simulink model "c00009M_harness"  (R2018a)
settings: Solver=FixedStepAuto  StartTime=0.0  StopTime=300  FixedStep=0.1  RelTol=1e-3
undefined symbols (not defined in the file): A1, hmax, PriorityTank, R1, R2, sigbuilder_block
(part 1 of 29)
settings Model: Creator=aarrieta  LastModifiedBy=umarkiegi

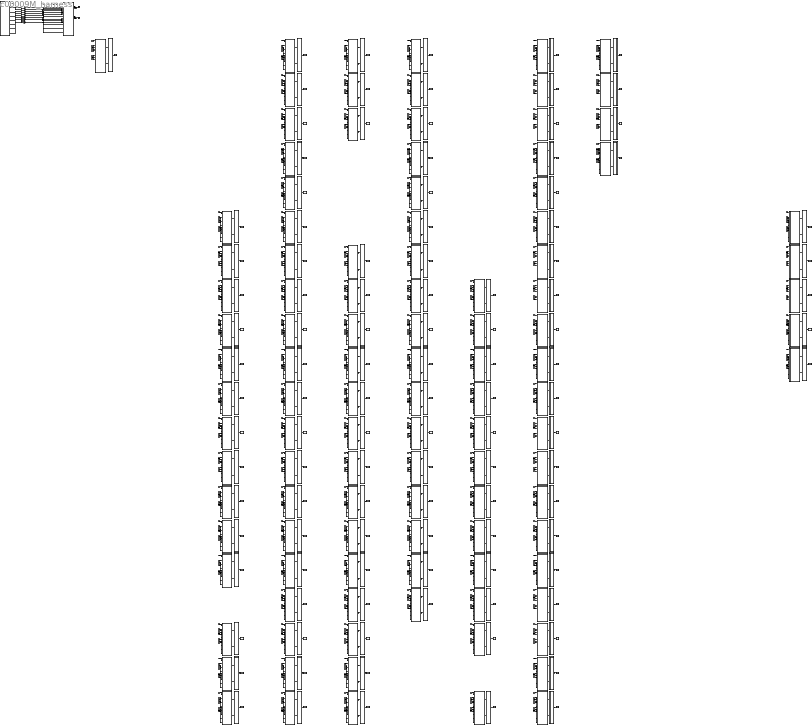
== system c00009M_harness ==
  CPSUT : Subsystem
  Eval : Subsystem
  Eval100 : Subsystem
  Eval101 : Subsystem
  Eval102 : Subsystem
  Eval103 : Subsystem
  Eval104 : Subsystem
  Eval105 : Subsystem
  Eval106 : Subsystem
  Eval107 : Subsystem
  Eval108 : Subsystem
  Eval109 : Subsystem
  Eval110 : Subsystem
  Eval111 : Subsystem
  Eval112 : Subsystem
  Eval113 : Subsystem
  Eval114 : Subsystem
  Eval115 : Subsystem
  Eval116 : Subsystem
  Eval127 : Subsystem
  Eval128 : Subsystem
  Eval129 : Subsystem
  Eval130 : Subsystem
  Eval131 : Subsystem
  Eval132 : Subsystem
  Eval133 : Subsystem
  Eval134 : Subsystem
  Eval135 : Subsystem
  Eval136 : Subsystem
  Eval137 : Subsystem
  Eval139 : Subsystem
  Eval140 : Subsystem
  Eval141 : Subsystem
  Eval142 : Subsystem
  Eval143 : Subsystem
  Eval144 : Subsystem
  Eval145 : Subsystem
  Eval146 : Subsystem
  Eval147 : Subsystem
  Eval148 : Subsystem
  Eval149 : Subsystem
  Eval150 : Subsystem
  Eval151 : Subsystem
  Eval152 : Subsystem
  Eval153 : Subsystem
  Eval154 : Subsystem
  Eval155 : Subsystem
  Eval156 : Subsystem
  Eval157 : Subsystem
  Eval158 : Subsystem
  Eval159 : Subsystem
  Eval160 : Subsystem
  Eval161 : Subsystem
  Eval162 : Subsystem
  Eval163 : Subsystem
  Eval225 : Subsystem
  Eval226 : Subsystem
  Eval227 : Subsystem
  Eval228 : Subsystem
  Eval229 : Subsystem
  Eval45 : Subsystem
  Eval46 : Subsystem
  Eval47 : Subsystem
  Eval48 : Subsystem
  Eval49 : Subsystem
  Eval50 : Subsystem
  Eval51 : Subsystem
  Eval52 : Subsystem
  Eval53 : Subsystem
  Eval54 : Subsystem
  Eval55 : Subsystem
  Eval57 : Subsystem
  Eval58 : Subsystem
  Eval59 : Subsystem
  Eval60 : Subsystem
  Eval61 : Subsystem
  Eval62 : Subsystem
  Eval63 : Subsystem
  Eval64 : Subsystem
  Eval65 : Subsystem
  Eval66 : Subsystem
  Eval67 : Subsystem
  Eval68 : Subsystem
  Eval69 : Subsystem
  Eval70 : Subsystem
  Eval71 : Subsystem
  Eval72 : Subsystem
  Eval73 : Subsystem
  Eval74 : Subsystem
  Eval75 : Subsystem
  Eval76 : Subsystem
  Eval77 : Subsystem
  Eval78 : Subsystem
  Eval79 : Subsystem
  Eval80 : Subsystem
  Eval81 : Subsystem
  Eval82 : Subsystem
  Eval86 : Subsystem
  Eval87 : Subsystem
  Eval88 : Subsystem
  Eval89 : Subsystem
  Eval90 : Subsystem
  Eval91 : Subsystem
  Eval92 : Subsystem
  Eval93 : Subsystem
  Eval94 : Subsystem
  Eval95 : Subsystem
  Eval96 : Subsystem
  Eval97 : Subsystem
  Eval98 : Subsystem
  Eval99 : Subsystem
  Inputs : Subsystem  Tag=STV Subsys  LoadFcn=sigbuilder_block('load');  StartFcn=sigbuilder_block('start');  StopFcn=sigbuilder_block('stop');  ClipboardFcn=sigbuilder_block('clipboard');  mask(Sigbuilder block){tuvar=[0:10]}
      mask init:
      | if ~strcmp(get_param(bdroot(gcb),'SimulationStatus'),'stopped'),tuvar = sigbuilder_block('maskInit'); end
      settings: CopyFcn=sigbuilder_block('copy');  DeleteFcn=sigbuilder_block('delete');  ModelCloseFcn=sigbuilder_block('modelClose');  PreSaveFcn=sigbuilder_block('preSave');  PauseFcn=sigbuilder_block('pause');  ContinueFcn=sigbuilder_block('continue');  NameChangeFcn=sigbuilder_block('namechange');  OpenFcn=sigbuilder_block('open',[276.75 163.5 675.75 486.75 ]);  CloseFcn=sigbuilder_block('close');
      mask Display: plot(0, 0, 100, 100,[2, 2, 32, 32, 2], [68, 8, 8, 68, 68],[32, 2], [38, 38], [32, 19, 2],[53, 60, 44], [32, 17, 17, 2],[16, 16, 31, 31]);txt = getActiveGroup(gcbh);text(2, 100, txt,'verticalAlignment', 'top');
  M001 : Subsystem
  M046 : Subsystem
  M047 : Subsystem
  M048 : Subsystem
  M049 : Subsystem
  M050 : Subsystem
  M051 : Subsystem
  M052 : Subsystem
  M053 : Subsystem
  M054 : Subsystem
  M055 : Subsystem
  M056 : Subsystem
  M058 : Subsystem
  M059 : Subsystem
  M060 : Subsystem
  M061 : Subsystem
  M062 : Subsystem
  M063 : Subsystem
  M064 : Subsystem
  M065 : Subsystem
  M066 : Subsystem
  M067 : Subsystem
  M068 : Subsystem
  M069 : Subsystem
  M070 : Subsystem
  M071 : Subsystem
  M072 : Subsystem
  M073 : Subsystem
  M074 : Subsystem
  M075 : Subsystem
  M076 : Subsystem
  M077 : Subsystem
  M078 : Subsystem
  M079 : Subsystem
  M080 : Subsystem
  M081 : Subsystem
  M082 : Subsystem
  M083 : Subsystem
  M087 : Subsystem
  M088 : Subsystem
  M089 : Subsystem
  M090 : Subsystem
  M091 : Subsystem
  M092 : Subsystem
  M093 : Subsystem
  M094 : Subsystem
  M095 : Subsystem
  M096 : Subsystem
  M097 : Subsystem
  M098 : Subsystem
  M099 : Subsystem
  M100 : Subsystem
  M101 : Subsystem
  M102 : Subsystem
  M103 : Subsystem
  M104 : Subsystem
  M105 : Subsystem
  M106 : Subsystem
  M107 : Subsystem
  M108 : Subsystem
  M109 : Subsystem
  M110 : Subsystem
  M111 : Subsystem
  M112 : Subsystem
  M113 : Subsystem
  M114 : Subsystem
  M115 : Subsystem
  M116 : Subsystem
  M117 : Subsystem
  M128 : Subsystem
  M129 : Subsystem
  M130 : Subsystem
  M131 : Subsystem
  M132 : Subsystem
  M133 : Subsystem
  M134 : Subsystem
  M135 : Subsystem
  M136 : Subsystem
  M137 : Subsystem
  M138 : Subsystem
  M140 : Subsystem
  M141 : Subsystem
  M142 : Subsystem
  M143 : Subsystem
  M144 : Subsystem
  M145 : Subsystem
  M146 : Subsystem
  M147 : Subsystem
  M148 : Subsystem
  M149 : Subsystem
  M150 : Subsystem
  M151 : Subsystem
  M152 : Subsystem
  M153 : Subsystem
  M154 : Subsystem
  M155 : Subsystem
  M156 : Subsystem
  M157 : Subsystem
  M158 : Subsystem
  M159 : Subsystem
  M160 : Subsystem
  M161 : Subsystem
  M162 : Subsystem
  M163 : Subsystem
  M164 : Subsystem
  M226 : Subsystem
  M227 : Subsystem
  M228 : Subsystem
  M229 : Subsystem
  M230 : Subsystem
  To Workspace : ToWorkspace  VariableName=mutant001  SampleTime=-1
  To Workspace100 : ToWorkspace  VariableName=mutant101  SampleTime=-1
  To Workspace101 : ToWorkspace  VariableName=mutant102  SampleTime=-1
  To Workspace102 : ToWorkspace  VariableName=mutant103  SampleTime=-1
  To Workspace103 : ToWorkspace  VariableName=mutant104  SampleTime=-1
  To Workspace104 : ToWorkspace  VariableName=mutant105  SampleTime=-1
  To Workspace105 : ToWorkspace  VariableName=mutant106  SampleTime=-1
  To Workspace106 : ToWorkspace  VariableName=mutant107  SampleTime=-1
  To Workspace107 : ToWorkspace  VariableName=mutant108  SampleTime=-1
  To Workspace108 : ToWorkspace  VariableName=mutant109  SampleTime=-1
  To Workspace109 : ToWorkspace  VariableName=mutant110  SampleTime=-1
  To Workspace110 : ToWorkspace  VariableName=mutant111  SampleTime=-1
  To Workspace111 : ToWorkspace  VariableName=mutant112  SampleTime=-1
  To Workspace112 : ToWorkspace  VariableName=mutant113  SampleTime=-1
  To Workspace113 : ToWorkspace  VariableName=mutant114  SampleTime=-1
  To Workspace114 : ToWorkspace  VariableName=mutant115  SampleTime=-1
  To Workspace115 : ToWorkspace  VariableName=mutant116  SampleTime=-1
  To Workspace116 : ToWorkspace  VariableName=mutant117  SampleTime=-1
  To Workspace127 : ToWorkspace  VariableName=mutant128  SampleTime=-1
  To Workspace128 : ToWorkspace  VariableName=mutant129  SampleTime=-1
  To Workspace129 : ToWorkspace  VariableName=mutant130  SampleTime=-1
  To Workspace130 : ToWorkspace  VariableName=mutant131  SampleTime=-1
  To Workspace131 : ToWorkspace  VariableName=mutant132  SampleTime=-1
  To Workspace132 : ToWorkspace  VariableName=mutant133  SampleTime=-1
  To Workspace133 : ToWorkspace  VariableName=mutant134  SampleTime=-1
  To Workspace134 : ToWorkspace  VariableName=mutant135  SampleTime=-1
  To Workspace135 : ToWorkspace  VariableName=mutant136  SampleTime=-1
  To Workspace136 : ToWorkspace  VariableName=mutant137  SampleTime=-1
  To Workspace137 : ToWorkspace  VariableName=mutant138  SampleTime=-1
  To Workspace139 : ToWorkspace  VariableName=mutant140  SampleTime=-1
  To Workspace140 : ToWorkspace  VariableName=mutant141  SampleTime=-1
  To Workspace141 : ToWorkspace  VariableName=mutant142  SampleTime=-1
  To Workspace142 : ToWorkspace  VariableName=mutant143  SampleTime=-1
  To Workspace143 : ToWorkspace  VariableName=mutant144  SampleTime=-1
  To Workspace144 : ToWorkspace  VariableName=mutant145  SampleTime=-1
  To Workspace145 : ToWorkspace  VariableName=mutant146  SampleTime=-1
  To Workspace146 : ToWorkspace  VariableName=mutant147  SampleTime=-1
  To Workspace147 : ToWorkspace  VariableName=mutant148  SampleTime=-1
  To Workspace148 : ToWorkspace  VariableName=mutant149  SampleTime=-1
  To Workspace149 : ToWorkspace  VariableName=mutant150  SampleTime=-1
  To Workspace150 : ToWorkspace  VariableName=mutant151  SampleTime=-1
  To Workspace151 : ToWorkspace  VariableName=mutant152  SampleTime=-1
  To Workspace152 : ToWorkspace  VariableName=mutant153  SampleTime=-1
  To Workspace153 : ToWorkspace  VariableName=mutant154  SampleTime=-1
  To Workspace154 : ToWorkspace  VariableName=mutant155  SampleTime=-1
  To Workspace155 : ToWorkspace  VariableName=mutant156  SampleTime=-1
  To Workspace156 : ToWorkspace  VariableName=mutant157  SampleTime=-1
  To Workspace157 : ToWorkspace  VariableName=mutant158  SampleTime=-1
  To Workspace158 : ToWorkspace  VariableName=mutant159  SampleTime=-1
  To Workspace159 : ToWorkspace  VariableName=mutant160  SampleTime=-1
  To Workspace160 : ToWorkspace  VariableName=mutant161  SampleTime=-1
  To Workspace161 : ToWorkspace  VariableName=mutant162  SampleTime=-1
  To Workspace162 : ToWorkspace  VariableName=mutant163  SampleTime=-1
  To Workspace163 : ToWorkspace  VariableName=mutant164  SampleTime=-1
  To Workspace225 : ToWorkspace  VariableName=mutant226  SampleTime=-1
  To Workspace226 : ToWorkspace  VariableName=mutant227  SampleTime=-1
  To Workspace227 : ToWorkspace  VariableName=mutant228  SampleTime=-1
  To Workspace228 : ToWorkspace  VariableName=mutant229  SampleTime=-1
  To Workspace229 : ToWorkspace  VariableName=mutant230  SampleTime=-1
  To Workspace45 : ToWorkspace  VariableName=mutant046  SampleTime=-1
  To Workspace46 : ToWorkspace  VariableName=mutant047  SampleTime=-1
  To Workspace47 : ToWorkspace  VariableName=mutant048  SampleTime=-1
  To Workspace48 : ToWorkspace  VariableName=mutant049  SampleTime=-1
  To Workspace49 : ToWorkspace  VariableName=mutant050  SampleTime=-1
  To Workspace50 : ToWorkspace  VariableName=mutant051  SampleTime=-1
  To Workspace51 : ToWorkspace  VariableName=mutant052  SampleTime=-1
  To Workspace52 : ToWorkspace  VariableName=mutant053  SampleTime=-1
  To Workspace53 : ToWorkspace  VariableName=mutant054  SampleTime=-1
  To Workspace54 : ToWorkspace  VariableName=mutant055  SampleTime=-1
  To Workspace55 : ToWorkspace  VariableName=mutant056  SampleTime=-1
  To Workspace57 : ToWorkspace  VariableName=mutant058  SampleTime=-1
  To Workspace58 : ToWorkspace  VariableName=mutant059  SampleTime=-1
  To Workspace59 : ToWorkspace  VariableName=mutant060  SampleTime=-1
  To Workspace60 : ToWorkspace  VariableName=mutant061  SampleTime=-1
  To Workspace61 : ToWorkspace  VariableName=mutant062  SampleTime=-1
  To Workspace62 : ToWorkspace  VariableName=mutant063  SampleTime=-1
  To Workspace63 : ToWorkspace  VariableName=mutant064  SampleTime=-1
  To Workspace64 : ToWorkspace  VariableName=mutant065  SampleTime=-1
  To Workspace65 : ToWorkspace  VariableName=mutant066  SampleTime=-1
  To Workspace66 : ToWorkspace  VariableName=mutant067  SampleTime=-1
  To Workspace67 : ToWorkspace  VariableName=mutant068  SampleTime=-1
  To Workspace68 : ToWorkspace  VariableName=mutant069  SampleTime=-1
  To Workspace69 : ToWorkspace  VariableName=mutant070  SampleTime=-1
  To Workspace70 : ToWorkspace  VariableName=mutant071  SampleTime=-1
  To Workspace71 : ToWorkspace  VariableName=mutant072  SampleTime=-1
  To Workspace72 : ToWorkspace  VariableName=mutant073  SampleTime=-1
  To Workspace73 : ToWorkspace  VariableName=mutant074  SampleTime=-1
  To Workspace74 : ToWorkspace  VariableName=mutant075  SampleTime=-1
  To Workspace75 : ToWorkspace  VariableName=mutant076  SampleTime=-1
  To Workspace76 : ToWorkspace  VariableName=mutant077  SampleTime=-1
  To Workspace77 : ToWorkspace  VariableName=mutant078  SampleTime=-1
  To Workspace78 : ToWorkspace  VariableName=mutant079  SampleTime=-1
  To Workspace79 : ToWorkspace  VariableName=mutant080  SampleTime=-1
  To Workspace80 : ToWorkspace  VariableName=mutant081  SampleTime=-1
  To Workspace81 : ToWorkspace  VariableName=mutant082  SampleTime=-1
  To Workspace82 : ToWorkspace  VariableName=mutant083  SampleTime=-1
  To Workspace86 : ToWorkspace  VariableName=mutant087  SampleTime=-1
  To Workspace87 : ToWorkspace  VariableName=mutant088  SampleTime=-1
  To Workspace88 : ToWorkspace  VariableName=mutant089  SampleTime=-1
  To Workspace89 : ToWorkspace  VariableName=mutant090  SampleTime=-1
  To Workspace90 : ToWorkspace  VariableName=mutant091  SampleTime=-1
  To Workspace91 : ToWorkspace  VariableName=mutant092  SampleTime=-1
  To Workspace92 : ToWorkspace  VariableName=mutant093  SampleTime=-1
  To Workspace93 : ToWorkspace  VariableName=mutant094  SampleTime=-1
  To Workspace94 : ToWorkspace  VariableName=mutant095  SampleTime=-1
  To Workspace95 : ToWorkspace  VariableName=mutant096  SampleTime=-1
  To Workspace96 : ToWorkspace  VariableName=mutant097  SampleTime=-1
  To Workspace97 : ToWorkspace  VariableName=mutant098  SampleTime=-1
  To Workspace98 : ToWorkspace  VariableName=mutant099  SampleTime=-1
  To Workspace99 : ToWorkspace  VariableName=mutant100  SampleTime=-1
  dtc_CT1 : DataTypeConversion
  dtc_CT2 : DataTypeConversion
  dtc_EB1 : DataTypeConversion
  dtc_EB2 : DataTypeConversion
  dtc_MR1 : DataTypeConversion
  dtc_MR2 : DataTypeConversion
  dtc_T1 : DataTypeConversion
  dtc_T2 : DataTypeConversion
  LL1 : Outport
  LL2 : Outport  Port=2
  tag scope: out1=global, out2=global
  wires:
  CPSUT/1(LL1) -> [out1], LL1/1
  CPSUT/2(LL2) -> [out2], LL2/1
  [in1] -> M001/1(CT1)
  [in4] -> M001/2(MR1)
  [in5] -> M001/3(T1)
  [in6] -> M001/4(EB1)
  [in7] -> M001/5(CT2)
  [in10] -> M001/6(MR2)
  [in11] -> M001/7(T2)
  [in12] -> M001/8(EB2)
  Eval/1(Out1) -> To Workspace/1
  M001/1(LL1) -> Eval/1(In1)
  M001/2(LL2) -> Eval/2(In2)
  [in1] -> M046/1(CT1)
  [in4] -> M046/2(MR1)
  [in5] -> M046/3(T1)
  [in6] -> M046/4(EB1)
  [in7] -> M046/5(CT2)
  [in10] -> M046/6(MR2)
  [in11] -> M046/7(T2)
  [in12] -> M046/8(EB2)
  M046/1(LL1) -> Eval45/1(In1)
  M046/2(LL2) -> Eval45/2(In2)
  Eval45/1(Out1) -> To Workspace45/1
  [in1] -> M047/1(CT1)
  [in4] -> M047/2(MR1)
  [in5] -> M047/3(T1)
  [in6] -> M047/4(EB1)
  [in7] -> M047/5(CT2)
  [in10] -> M047/6(MR2)
  [in11] -> M047/7(T2)
  [in12] -> M047/8(EB2)
  M047/1(LL1) -> Eval46/1(In1)
  M047/2(LL2) -> Eval46/2(In2)
  Eval46/1(Out1) -> To Workspace46/1
  [in1] -> M048/1(CT1)
  [in4] -> M048/2(MR1)
  [in5] -> M048/3(T1)
  [in6] -> M048/4(EB1)
  [in7] -> M048/5(CT2)
  [in10] -> M048/6(MR2)
  [in11] -> M048/7(T2)
  [in12] -> M048/8(EB2)
  M048/1(LL1) -> Eval47/1(In1)
  M048/2(LL2) -> Eval47/2(In2)
  Eval47/1(Out1) -> To Workspace47/1
  [in1] -> M049/1(CT1)
  [in4] -> M049/2(MR1)
  [in5] -> M049/3(T1)
  [in6] -> M049/4(EB1)
  [in7] -> M049/5(CT2)
  [in10] -> M049/6(MR2)
  [in11] -> M049/7(T2)
  [in12] -> M049/8(EB2)
  M049/1(LL1) -> Eval48/1(In1)
  M049/2(LL2) -> Eval48/2(In2)
  Eval48/1(Out1) -> To Workspace48/1
  [in1] -> M050/1(CT1)
  [in4] -> M050/2(MR1)
  [in5] -> M050/3(T1)
  [in6] -> M050/4(EB1)
  [in7] -> M050/5(CT2)
  [in10] -> M050/6(MR2)
  [in11] -> M050/7(T2)
  [in12] -> M050/8(EB2)
  M050/1(LL1) -> Eval49/1(In1)
  M050/2(LL2) -> Eval49/2(In2)
  Eval49/1(Out1) -> To Workspace49/1
  [in1] -> M051/1(CT1)
  [in4] -> M051/2(MR1)
  [in5] -> M051/3(T1)
  [in6] -> M051/4(EB1)
  [in7] -> M051/5(CT2)
  [in10] -> M051/6(MR2)
  [in11] -> M051/7(T2)
  [in12] -> M051/8(EB2)
  M051/1(LL1) -> Eval50/1(In1)
  M051/2(LL2) -> Eval50/2(In2)
  Eval50/1(Out1) -> To Workspace50/1
  [in1] -> M052/1(CT1)
  [in4] -> M052/2(MR1)
  [in5] -> M052/3(T1)
  [in6] -> M052/4(EB1)
  [in7] -> M052/5(CT2)
  [in10] -> M052/6(MR2)
  [in11] -> M052/7(T2)
  [in12] -> M052/8(EB2)
  M052/1(LL1) -> Eval51/1(In1)
  M052/2(LL2) -> Eval51/2(In2)
  Eval51/1(Out1) -> To Workspace51/1
  [in1] -> M053/1(CT1)
  [in4] -> M053/2(MR1)
  [in5] -> M053/3(T1)
  [in6] -> M053/4(EB1)
  [in7] -> M053/5(CT2)
  [in10] -> M053/6(MR2)
  [in11] -> M053/7(T2)
  [in12] -> M053/8(EB2)
  M053/1(LL1) -> Eval52/1(In1)
  M053/2(LL2) -> Eval52/2(In2)
  Eval52/1(Out1) -> To Workspace52/1
  [in1] -> M054/1(CT1)
  [in4] -> M054/2(MR1)
  [in5] -> M054/3(T1)
  [in6] -> M054/4(EB1)
  [in7] -> M054/5(CT2)
  [in10] -> M054/6(MR2)
  [in11] -> M054/7(T2)
  [in12] -> M054/8(EB2)
  M054/1(LL1) -> Eval53/1(In1)
  M054/2(LL2) -> Eval53/2(In2)
  Eval53/1(Out1) -> To Workspace53/1
  [in1] -> M055/1(CT1)
  [in4] -> M055/2(MR1)
  [in5] -> M055/3(T1)
  [in6] -> M055/4(EB1)
  [in7] -> M055/5(CT2)
  [in10] -> M055/6(MR2)
  [in11] -> M055/7(T2)
  [in12] -> M055/8(EB2)
  M055/1(LL1) -> Eval54/1(In1)
  M055/2(LL2) -> Eval54/2(In2)
  Eval54/1(Out1) -> To Workspace54/1
  [in1] -> M056/1(CT1)
  [in4] -> M056/2(MR1)
  [in5] -> M056/3(T1)
  [in6] -> M056/4(EB1)
  [in7] -> M056/5(CT2)
  [in10] -> M056/6(MR2)
  [in11] -> M056/7(T2)
  [in12] -> M056/8(EB2)
  M056/1(LL1) -> Eval55/1(In1)
  M056/2(LL2) -> Eval55/2(In2)
  Eval55/1(Out1) -> To Workspace55/1
  [in1] -> M058/1(CT1)
  [in4] -> M058/2(MR1)
  [in5] -> M058/3(T1)
  [in6] -> M058/4(EB1)
  [in7] -> M058/5(CT2)
  [in10] -> M058/6(MR2)
  [in11] -> M058/7(T2)
  [in12] -> M058/8(EB2)
  M058/1(LL1) -> Eval57/1(In1)
  M058/2(LL2) -> Eval57/2(In2)
  Eval57/1(Out1) -> To Workspace57/1
  [in1] -> M059/1(CT1)
  [in4] -> M059/2(MR1)
  [in5] -> M059/3(T1)
  [in6] -> M059/4(EB1)
  [in7] -> M059/5(CT2)
  [in10] -> M059/6(MR2)
  [in11] -> M059/7(T2)
  [in12] -> M059/8(EB2)
  M059/1(LL1) -> Eval58/1(In1)
  M059/2(LL2) -> Eval58/2(In2)
  Eval58/1(Out1) -> To Workspace58/1
  [in1] -> M060/1(CT1)
  [in4] -> M060/2(MR1)
  [in5] -> M060/3(T1)
  [in6] -> M060/4(EB1)
  [in7] -> M060/5(CT2)
  [in10] -> M060/6(MR2)
  [in11] -> M060/7(T2)
  [in12] -> M060/8(EB2)
  M060/1(LL1) -> Eval59/1(In1)
  M060/2(LL2) -> Eval59/2(In2)
  Eval59/1(Out1) -> To Workspace59/1
  [in1] -> M061/1(CT1)
  [in4] -> M061/2(MR1)
  [in5] -> M061/3(T1)
  [in6] -> M061/4(EB1)
  [in7] -> M061/5(CT2)
  [in10] -> M061/6(MR2)
  [in11] -> M061/7(T2)
  [in12] -> M061/8(EB2)
  M061/1(LL1) -> Eval60/1(In1)
  M061/2(LL2) -> Eval60/2(In2)
  Eval60/1(Out1) -> To Workspace60/1
  [in1] -> M062/1(CT1)
  [in4] -> M062/2(MR1)
  [in5] -> M062/3(T1)
  [in6] -> M062/4(EB1)
  [in7] -> M062/5(CT2)
  [in10] -> M062/6(MR2)
  [in11] -> M062/7(T2)
  [in12] -> M062/8(EB2)
  M062/1(LL1) -> Eval61/1(In1)
  M062/2(LL2) -> Eval61/2(In2)
  Eval61/1(Out1) -> To Workspace61/1
  [in1] -> M063/1(CT1)
  [in4] -> M063/2(MR1)
  [in5] -> M063/3(T1)
  [in6] -> M063/4(EB1)
  [in7] -> M063/5(CT2)
  [in10] -> M063/6(MR2)
  [in11] -> M063/7(T2)
  [in12] -> M063/8(EB2)
  M063/1(LL1) -> Eval62/1(In1)
  M063/2(LL2) -> Eval62/2(In2)
  Eval62/1(Out1) -> To Workspace62/1
  [in1] -> M064/1(CT1)
  [in4] -> M064/2(MR1)
  [in5] -> M064/3(T1)
  [in6] -> M064/4(EB1)
  [in7] -> M064/5(CT2)
  [in10] -> M064/6(MR2)
  [in11] -> M064/7(T2)
  [in12] -> M064/8(EB2)
  M064/1(LL1) -> Eval63/1(In1)
  M064/2(LL2) -> Eval63/2(In2)
  Eval63/1(Out1) -> To Workspace63/1
  [in1] -> M065/1(CT1)
  [in4] -> M065/2(MR1)
  [in5] -> M065/3(T1)
  [in6] -> M065/4(EB1)
  [in7] -> M065/5(CT2)
  [in10] -> M065/6(MR2)
  [in11] -> M065/7(T2)
  [in12] -> M065/8(EB2)
  M065/1(LL1) -> Eval64/1(In1)
  M065/2(LL2) -> Eval64/2(In2)
  Eval64/1(Out1) -> To Workspace64/1
  [in1] -> M066/1(CT1)
  [in4] -> M066/2(MR1)
  [in5] -> M066/3(T1)
  [in6] -> M066/4(EB1)
  [in7] -> M066/5(CT2)
  [in10] -> M066/6(MR2)
  [in11] -> M066/7(T2)
  [in12] -> M066/8(EB2)
  M066/1(LL1) -> Eval65/1(In1)
  M066/2(LL2) -> Eval65/2(In2)
  Eval65/1(Out1) -> To Workspace65/1
  [in1] -> M067/1(CT1)
  [in4] -> M067/2(MR1)
  [in5] -> M067/3(T1)
  [in6] -> M067/4(EB1)
  [in7] -> M067/5(CT2)
  [in10] -> M067/6(MR2)
  [in11] -> M067/7(T2)
  [in12] -> M067/8(EB2)
  M067/1(LL1) -> Eval66/1(In1)
  M067/2(LL2) -> Eval66/2(In2)
  Eval66/1(Out1) -> To Workspace66/1
  [in1] -> M068/1(CT1)
  [in4] -> M068/2(MR1)
  [in5] -> M068/3(T1)
  [in6] -> M068/4(EB1)
  [in7] -> M068/5(CT2)
  [in10] -> M068/6(MR2)
  [in11] -> M068/7(T2)
  [in12] -> M068/8(EB2)
  M068/1(LL1) -> Eval67/1(In1)
  M068/2(LL2) -> Eval67/2(In2)
  Eval67/1(Out1) -> To Workspace67/1
  [in1] -> M069/1(CT1)
  [in4] -> M069/2(MR1)
  [in5] -> M069/3(T1)
  [in6] -> M069/4(EB1)
  [in7] -> M069/5(CT2)
  [in10] -> M069/6(MR2)
  [in11] -> M069/7(T2)
  [in12] -> M069/8(EB2)
  M069/1(LL1) -> Eval68/1(In1)
  M069/2(LL2) -> Eval68/2(In2)
  Eval68/1(Out1) -> To Workspace68/1
  [in1] -> M070/1(CT1)
  [in4] -> M070/2(MR1)
  [in5] -> M070/3(T1)
  [in6] -> M070/4(EB1)
  [in7] -> M070/5(CT2)
  [in10] -> M070/6(MR2)
  [in11] -> M070/7(T2)
  [in12] -> M070/8(EB2)
  M070/1(LL1) -> Eval69/1(In1)
  M070/2(LL2) -> Eval69/2(In2)
  Eval69/1(Out1) -> To Workspace69/1
  [in1] -> M071/1(CT1)
  [in4] -> M071/2(MR1)
  [in5] -> M071/3(T1)
  [in6] -> M071/4(EB1)
  [in7] -> M071/5(CT2)
  [in10] -> M071/6(MR2)
  [in11] -> M071/7(T2)
  [in12] -> M071/8(EB2)
  M071/1(LL1) -> Eval70/1(In1)
  M071/2(LL2) -> Eval70/2(In2)
  Eval70/1(Out1) -> To Workspace70/1
  [in1] -> M072/1(CT1)
  [in4] -> M072/2(MR1)
  [in5] -> M072/3(T1)
  [in6] -> M072/4(EB1)
  [in7] -> M072/5(CT2)
  [in10] -> M072/6(MR2)
  [in11] -> M072/7(T2)
  [in12] -> M072/8(EB2)
  M072/1(LL1) -> Eval71/1(In1)
  M072/2(LL2) -> Eval71/2(In2)
  Eval71/1(Out1) -> To Workspace71/1
  [in1] -> M073/1(CT1)
  [in4] -> M073/2(MR1)
  [in5] -> M073/3(T1)
  [in6] -> M073/4(EB1)
  [in7] -> M073/5(CT2)
  [in10] -> M073/6(MR2)
  [in11] -> M073/7(T2)
  [in12] -> M073/8(EB2)
  M073/1(LL1) -> Eval72/1(In1)
  M073/2(LL2) -> Eval72/2(In2)
  Eval72/1(Out1) -> To Workspace72/1
  [in1] -> M074/1(CT1)
  [in4] -> M074/2(MR1)
  [in5] -> M074/3(T1)
  [in6] -> M074/4(EB1)
  [in7] -> M074/5(CT2)
  [in10] -> M074/6(MR2)
  [in11] -> M074/7(T2)
  [in12] -> M074/8(EB2)
  M074/1(LL1) -> Eval73/1(In1)
  M074/2(LL2) -> Eval73/2(In2)
  Eval73/1(Out1) -> To Workspace73/1
  [in1] -> M075/1(CT1)
  [in4] -> M075/2(MR1)
  [in5] -> M075/3(T1)
  [in6] -> M075/4(EB1)
  [in7] -> M075/5(CT2)
  [in10] -> M075/6(MR2)
  [in11] -> M075/7(T2)
  [in12] -> M075/8(EB2)
  M075/1(LL1) -> Eval74/1(In1)
  M075/2(LL2) -> Eval74/2(In2)
  Eval74/1(Out1) -> To Workspace74/1
  [in1] -> M076/1(CT1)
  [in4] -> M076/2(MR1)
  [in5] -> M076/3(T1)
  [in6] -> M076/4(EB1)
  [in7] -> M076/5(CT2)
  [in10] -> M076/6(MR2)
  [in11] -> M076/7(T2)
  [in12] -> M076/8(EB2)
  M076/1(LL1) -> Eval75/1(In1)
  M076/2(LL2) -> Eval75/2(In2)
  Eval75/1(Out1) -> To Workspace75/1
  [in1] -> M077/1(CT1)
  [in4] -> M077/2(MR1)
  [in5] -> M077/3(T1)
  [in6] -> M077/4(EB1)
  [in7] -> M077/5(CT2)
  [in10] -> M077/6(MR2)
  [in11] -> M077/7(T2)
  [in12] -> M077/8(EB2)
  M077/1(LL1) -> Eval76/1(In1)
  M077/2(LL2) -> Eval76/2(In2)
  Eval76/1(Out1) -> To Workspace76/1
  [in1] -> M078/1(CT1)
  [in4] -> M078/2(MR1)
  [in5] -> M078/3(T1)
  [in6] -> M078/4(EB1)
  [in7] -> M078/5(CT2)
  [in10] -> M078/6(MR2)
  [in11] -> M078/7(T2)
  [in12] -> M078/8(EB2)
  M078/1(LL1) -> Eval77/1(In1)
  M078/2(LL2) -> Eval77/2(In2)
  Eval77/1(Out1) -> To Workspace77/1
  [in1] -> M079/1(CT1)
  [in4] -> M079/2(MR1)
  [in5] -> M079/3(T1)
  [in6] -> M079/4(EB1)
  [in7] -> M079/5(CT2)
  [in10] -> M079/6(MR2)
  [in11] -> M079/7(T2)
  [in12] -> M079/8(EB2)
  M079/1(LL1) -> Eval78/1(In1)
  M079/2(LL2) -> Eval78/2(In2)
  Eval78/1(Out1) -> To Workspace78/1
  [in1] -> M080/1(CT1)
  [in4] -> M080/2(MR1)
  [in5] -> M080/3(T1)
  [in6] -> M080/4(EB1)
  [in7] -> M080/5(CT2)
  [in10] -> M080/6(MR2)
  [in11] -> M080/7(T2)
  [in12] -> M080/8(EB2)
  M080/1(LL1) -> Eval79/1(In1)
  M080/2(LL2) -> Eval79/2(In2)
  Eval79/1(Out1) -> To Workspace79/1
  [in1] -> M081/1(CT1)
  [in4] -> M081/2(MR1)
  [in5] -> M081/3(T1)
  [in6] -> M081/4(EB1)
  [in7] -> M081/5(CT2)
  [in10] -> M081/6(MR2)
  [in11] -> M081/7(T2)
  [in12] -> M081/8(EB2)
  M081/1(LL1) -> Eval80/1(In1)
  M081/2(LL2) -> Eval80/2(In2)
  Eval80/1(Out1) -> To Workspace80/1
  [in1] -> M082/1(CT1)
  [in4] -> M082/2(MR1)
  [in5] -> M082/3(T1)
  [in6] -> M082/4(EB1)
  [in7] -> M082/5(CT2)
  [in10] -> M082/6(MR2)
  [in11] -> M082/7(T2)
  [in12] -> M082/8(EB2)
  M082/1(LL1) -> Eval81/1(In1)
  M082/2(LL2) -> Eval81/2(In2)
  Eval81/1(Out1) -> To Workspace81/1
  [in1] -> M083/1(CT1)
  [in4] -> M083/2(MR1)
  [in5] -> M083/3(T1)
  [in6] -> M083/4(EB1)
  [in7] -> M083/5(CT2)
  [in10] -> M083/6(MR2)
  [in11] -> M083/7(T2)
  [in12] -> M083/8(EB2)
  M083/1(LL1) -> Eval82/1(In1)
  M083/2(LL2) -> Eval82/2(In2)
  Eval82/1(Out1) -> To Workspace82/1
  [in1] -> M087/1(CT1)
  [in4] -> M087/2(MR1)
  [in5] -> M087/3(T1)
  [in6] -> M087/4(EB1)
  [in7] -> M087/5(CT2)
  [in10] -> M087/6(MR2)
  [in11] -> M087/7(T2)
  [in12] -> M087/8(EB2)
  M087/1(LL1) -> Eval86/1(In1)
  M087/2(LL2) -> Eval86/2(In2)
  Eval86/1(Out1) -> To Workspace86/1
  [in1] -> M088/1(CT1)
  [in4] -> M088/2(MR1)
  [in5] -> M088/3(T1)
  [in6] -> M088/4(EB1)
  [in7] -> M088/5(CT2)
  [in10] -> M088/6(MR2)
  [in11] -> M088/7(T2)
  [in12] -> M088/8(EB2)
  M088/1(LL1) -> Eval87/1(In1)
  M088/2(LL2) -> Eval87/2(In2)
  Eval87/1(Out1) -> To Workspace87/1
  [in1] -> M089/1(CT1)
  [in4] -> M089/2(MR1)
  [in5] -> M089/3(T1)
  [in6] -> M089/4(EB1)
  [in7] -> M089/5(CT2)
  [in10] -> M089/6(MR2)
  [in11] -> M089/7(T2)
  [in12] -> M089/8(EB2)
  M089/1(LL1) -> Eval88/1(In1)
  M089/2(LL2) -> Eval88/2(In2)
  Eval88/1(Out1) -> To Workspace88/1
  [in1] -> M090/1(CT1)
  [in4] -> M090/2(MR1)
  [in5] -> M090/3(T1)
  [in6] -> M090/4(EB1)
  [in7] -> M090/5(CT2)
  [in10] -> M090/6(MR2)
  [in11] -> M090/7(T2)
  [in12] -> M090/8(EB2)
  M090/1(LL1) -> Eval89/1(In1)
  M090/2(LL2) -> Eval89/2(In2)
  Eval89/1(Out1) -> To Workspace89/1
  [in1] -> M091/1(CT1)
  [in4] -> M091/2(MR1)
  [in5] -> M091/3(T1)
  [in6] -> M091/4(EB1)
  [in7] -> M091/5(CT2)
  [in10] -> M091/6(MR2)
  [in11] -> M091/7(T2)
  [in12] -> M091/8(EB2)
  M091/1(LL1) -> Eval90/1(In1)
  M091/2(LL2) -> Eval90/2(In2)
  Eval90/1(Out1) -> To Workspace90/1
  [in1] -> M092/1(CT1)
  [in4] -> M092/2(MR1)
  [in5] -> M092/3(T1)
  [in6] -> M092/4(EB1)
  [in7] -> M092/5(CT2)
  [in10] -> M092/6(MR2)
  [in11] -> M092/7(T2)
  [in12] -> M092/8(EB2)
  M092/1(LL1) -> Eval91/1(In1)
  M092/2(LL2) -> Eval91/2(In2)
  Eval91/1(Out1) -> To Workspace91/1
  [in1] -> M093/1(CT1)
  [in4] -> M093/2(MR1)
  [in5] -> M093/3(T1)
  [in6] -> M093/4(EB1)
  [in7] -> M093/5(CT2)
  [in10] -> M093/6(MR2)
  [in11] -> M093/7(T2)
  [in12] -> M093/8(EB2)
  M093/1(LL1) -> Eval92/1(In1)
  M093/2(LL2) -> Eval92/2(In2)
  Eval92/1(Out1) -> To Workspace92/1
  [in1] -> M094/1(CT1)
  [in4] -> M094/2(MR1)
  [in5] -> M094/3(T1)
  [in6] -> M094/4(EB1)
  [in7] -> M094/5(CT2)
  [in10] -> M094/6(MR2)
  [in11] -> M094/7(T2)
  [in12] -> M094/8(EB2)
  M094/1(LL1) -> Eval93/1(In1)
  M094/2(LL2) -> Eval93/2(In2)
  Eval93/1(Out1) -> To Workspace93/1
  [in1] -> M095/1(CT1)
  [in4] -> M095/2(MR1)
  [in5] -> M095/3(T1)
  [in6] -> M095/4(EB1)
  [in7] -> M095/5(CT2)
  [in10] -> M095/6(MR2)
  [in11] -> M095/7(T2)
  [in12] -> M095/8(EB2)
  M095/1(LL1) -> Eval94/1(In1)
  M095/2(LL2) -> Eval94/2(In2)
  Eval94/1(Out1) -> To Workspace94/1
  [in1] -> M096/1(CT1)
  [in4] -> M096/2(MR1)
  [in5] -> M096/3(T1)
  [in6] -> M096/4(EB1)
  [in7] -> M096/5(CT2)
  [in10] -> M096/6(MR2)
  [in11] -> M096/7(T2)
  [in12] -> M096/8(EB2)
  M096/1(LL1) -> Eval95/1(In1)
  M096/2(LL2) -> Eval95/2(In2)
  Eval95/1(Out1) -> To Workspace95/1
  [in1] -> M097/1(CT1)
  [in4] -> M097/2(MR1)
  [in5] -> M097/3(T1)
  [in6] -> M097/4(EB1)
  [in7] -> M097/5(CT2)
  [in10] -> M097/6(MR2)
  [in11] -> M097/7(T2)
  [in12] -> M097/8(EB2)
  M097/1(LL1) -> Eval96/1(In1)
  M097/2(LL2) -> Eval96/2(In2)
  Eval96/1(Out1) -> To Workspace96/1
  [in1] -> M098/1(CT1)
  [in4] -> M098/2(MR1)
  [in5] -> M098/3(T1)
  [in6] -> M098/4(EB1)
  [in7] -> M098/5(CT2)
  [in10] -> M098/6(MR2)
  [in11] -> M098/7(T2)
  [in12] -> M098/8(EB2)
  M098/1(LL1) -> Eval97/1(In1)
  M098/2(LL2) -> Eval97/2(In2)
  Eval97/1(Out1) -> To Workspace97/1
  [in1] -> M099/1(CT1)
  [in4] -> M099/2(MR1)
  [in5] -> M099/3(T1)
  [in6] -> M099/4(EB1)
  [in7] -> M099/5(CT2)
  [in10] -> M099/6(MR2)
  [in11] -> M099/7(T2)
  [in12] -> M099/8(EB2)
  M099/1(LL1) -> Eval98/1(In1)
  M099/2(LL2) -> Eval98/2(In2)
  Eval98/1(Out1) -> To Workspace98/1
  [in1] -> M100/1(CT1)
  [in4] -> M100/2(MR1)
  [in5] -> M100/3(T1)
  [in6] -> M100/4(EB1)
  [in7] -> M100/5(CT2)
  [in10] -> M100/6(MR2)
  [in11] -> M100/7(T2)
  [in12] -> M100/8(EB2)
  M100/1(LL1) -> Eval99/1(In1)
  M100/2(LL2) -> Eval99/2(In2)
  Eval99/1(Out1) -> To Workspace99/1
  [in1] -> M101/1(CT1)
  [in4] -> M101/2(MR1)
  [in5] -> M101/3(T1)
  [in6] -> M101/4(EB1)
  [in7] -> M101/5(CT2)
  [in10] -> M101/6(MR2)
  [in11] -> M101/7(T2)
  [in12] -> M101/8(EB2)
  M101/1(LL1) -> Eval100/1(In1)
  M101/2(LL2) -> Eval100/2(In2)
  Eval100/1(Out1) -> To Workspace100/1
  [in1] -> M102/1(CT1)
  [in4] -> M102/2(MR1)
  [in5] -> M102/3(T1)
  [in6] -> M102/4(EB1)
  [in7] -> M102/5(CT2)
  [in10] -> M102/6(MR2)
  [in11] -> M102/7(T2)
  [in12] -> M102/8(EB2)
  M102/1(LL1) -> Eval101/1(In1)
  M102/2(LL2) -> Eval101/2(In2)
  Eval101/1(Out1) -> To Workspace101/1
  [in1] -> M103/1(CT1)
  [in4] -> M103/2(MR1)
  [in5] -> M103/3(T1)
  [in6] -> M103/4(EB1)
  [in7] -> M103/5(CT2)
  [in10] -> M103/6(MR2)
  [in11] -> M103/7(T2)
  [in12] -> M103/8(EB2)
  M103/1(LL1) -> Eval102/1(In1)
  M103/2(LL2) -> Eval102/2(In2)
  Eval102/1(Out1) -> To Workspace102/1
  [in1] -> M104/1(CT1)
  [in4] -> M104/2(MR1)
  [in5] -> M104/3(T1)
  [in6] -> M104/4(EB1)
  [in7] -> M104/5(CT2)
  [in10] -> M104/6(MR2)
  [in11] -> M104/7(T2)
  [in12] -> M104/8(EB2)
  M104/1(LL1) -> Eval103/1(In1)
  M104/2(LL2) -> Eval103/2(In2)
  Eval103/1(Out1) -> To Workspace103/1
  [in1] -> M105/1(CT1)
  [in4] -> M105/2(MR1)
  [in5] -> M105/3(T1)
  [in6] -> M105/4(EB1)
  [in7] -> M105/5(CT2)
  [in10] -> M105/6(MR2)
  [in11] -> M105/7(T2)
  [in12] -> M105/8(EB2)
  M105/1(LL1) -> Eval104/1(In1)
  M105/2(LL2) -> Eval104/2(In2)
  Eval104/1(Out1) -> To Workspace104/1
  [in1] -> M106/1(CT1)
  [in4] -> M106/2(MR1)
  [in5] -> M106/3(T1)
  [in6] -> M106/4(EB1)
  [in7] -> M106/5(CT2)
  [in10] -> M106/6(MR2)
  [in11] -> M106/7(T2)
  [in12] -> M106/8(EB2)
  M106/1(LL1) -> Eval105/1(In1)
  M106/2(LL2) -> Eval105/2(In2)
  Eval105/1(Out1) -> To Workspace105/1
  [in1] -> M107/1(CT1)
  [in4] -> M107/2(MR1)
  [in5] -> M107/3(T1)
  [in6] -> M107/4(EB1)
  [in7] -> M107/5(CT2)
  [in10] -> M107/6(MR2)
  [in11] -> M107/7(T2)
  [in12] -> M107/8(EB2)
  M107/1(LL1) -> Eval106/1(In1)
  M107/2(LL2) -> Eval106/2(In2)
  Eval106/1(Out1) -> To Workspace106/1
  [in1] -> M108/1(CT1)
  [in4] -> M108/2(MR1)
  [in5] -> M108/3(T1)
  [in6] -> M108/4(EB1)
  [in7] -> M108/5(CT2)
  [in10] -> M108/6(MR2)
  [in11] -> M108/7(T2)
  [in12] -> M108/8(EB2)
  M108/1(LL1) -> Eval107/1(In1)
  M108/2(LL2) -> Eval107/2(In2)
  Eval107/1(Out1) -> To Workspace107/1
  [in1] -> M109/1(CT1)
  [in4] -> M109/2(MR1)
  [in5] -> M109/3(T1)
  [in6] -> M109/4(EB1)
  [in7] -> M109/5(CT2)
  [in10] -> M109/6(MR2)
  [in11] -> M109/7(T2)
  [in12] -> M109/8(EB2)
  M109/1(LL1) -> Eval108/1(In1)
  M109/2(LL2) -> Eval108/2(In2)
  Eval108/1(Out1) -> To Workspace108/1
  [in1] -> M110/1(CT1)
  [in4] -> M110/2(MR1)
  [in5] -> M110/3(T1)
  [in6] -> M110/4(EB1)
  [in7] -> M110/5(CT2)
  [in10] -> M110/6(MR2)
  [in11] -> M110/7(T2)
  [in12] -> M110/8(EB2)
  M110/1(LL1) -> Eval109/1(In1)
  M110/2(LL2) -> Eval109/2(In2)
  Eval109/1(Out1) -> To Workspace109/1
  [in1] -> M111/1(CT1)
  [in4] -> M111/2(MR1)
  [in5] -> M111/3(T1)
  [in6] -> M111/4(EB1)
  [in7] -> M111/5(CT2)
  [in10] -> M111/6(MR2)
  [in11] -> M111/7(T2)
  [in12] -> M111/8(EB2)
  M111/1(LL1) -> Eval110/1(In1)
  M111/2(LL2) -> Eval110/2(In2)
  Eval110/1(Out1) -> To Workspace110/1
  [in1] -> M112/1(CT1)
  [in4] -> M112/2(MR1)
  [in5] -> M112/3(T1)
  [in6] -> M112/4(EB1)
  [in7] -> M112/5(CT2)
  [in10] -> M112/6(MR2)
  [in11] -> M112/7(T2)
  [in12] -> M112/8(EB2)
  M112/1(LL1) -> Eval111/1(In1)
  M112/2(LL2) -> Eval111/2(In2)
  Eval111/1(Out1) -> To Workspace111/1
  [in1] -> M113/1(CT1)
  [in4] -> M113/2(MR1)
  [in5] -> M113/3(T1)
  [in6] -> M113/4(EB1)
  [in7] -> M113/5(CT2)
  [in10] -> M113/6(MR2)
  [in11] -> M113/7(T2)
  [in12] -> M113/8(EB2)
  M113/1(LL1) -> Eval112/1(In1)
  M113/2(LL2) -> Eval112/2(In2)
  Eval112/1(Out1) -> To Workspace112/1
  [in1] -> M114/1(CT1)
  [in4] -> M114/2(MR1)
  [in5] -> M114/3(T1)
  [in6] -> M114/4(EB1)
  [in7] -> M114/5(CT2)
  [in10] -> M114/6(MR2)
  [in11] -> M114/7(T2)
  [in12] -> M114/8(EB2)
  M114/1(LL1) -> Eval113/1(In1)
  M114/2(LL2) -> Eval113/2(In2)
  Eval113/1(Out1) -> To Workspace113/1
  [in1] -> M115/1(CT1)
  [in4] -> M115/2(MR1)
  [in5] -> M115/3(T1)
  [in6] -> M115/4(EB1)
  [in7] -> M115/5(CT2)
  [in10] -> M115/6(MR2)
  [in11] -> M115/7(T2)
  [in12] -> M115/8(EB2)
  M115/1(LL1) -> Eval114/1(In1)
  M115/2(LL2) -> Eval114/2(In2)
  Eval114/1(Out1) -> To Workspace114/1
  [in1] -> M116/1(CT1)
  [in4] -> M116/2(MR1)
  [in5] -> M116/3(T1)
  [in6] -> M116/4(EB1)
  [in7] -> M116/5(CT2)
  [in10] -> M116/6(MR2)
  [in11] -> M116/7(T2)
  [in12] -> M116/8(EB2)
  M116/1(LL1) -> Eval115/1(In1)
  M116/2(LL2) -> Eval115/2(In2)
  Eval115/1(Out1) -> To Workspace115/1
  [in1] -> M117/1(CT1)
  [in4] -> M117/2(MR1)
  [in5] -> M117/3(T1)
  [in6] -> M117/4(EB1)
  [in7] -> M117/5(CT2)
  [in10] -> M117/6(MR2)
  [in11] -> M117/7(T2)
  [in12] -> M117/8(EB2)
  M117/1(LL1) -> Eval116/1(In1)
  M117/2(LL2) -> Eval116/2(In2)
  Eval116/1(Out1) -> To Workspace116/1
  [in1] -> M128/1(CT1)
  [in4] -> M128/2(MR1)
  [in5] -> M128/3(T1)
  [in6] -> M128/4(EB1)
  [in7] -> M128/5(CT2)
  [in10] -> M128/6(MR2)
  [in11] -> M128/7(T2)
  [in12] -> M128/8(EB2)
  M128/1(LL1) -> Eval127/1(In1)
  M128/2(LL2) -> Eval127/2(In2)
  Eval127/1(Out1) -> To Workspace127/1
  [in1] -> M129/1(CT1)
  [in4] -> M129/2(MR1)
  [in5] -> M129/3(T1)
  [in6] -> M129/4(EB1)
  [in7] -> M129/5(CT2)
  [in10] -> M129/6(MR2)
  [in11] -> M129/7(T2)
  [in12] -> M129/8(EB2)
  M129/1(LL1) -> Eval128/1(In1)
  M129/2(LL2) -> Eval128/2(In2)
  Eval128/1(Out1) -> To Workspace128/1
  [in1] -> M130/1(CT1)
  [in4] -> M130/2(MR1)
  [in5] -> M130/3(T1)
  [in6] -> M130/4(EB1)
  [in7] -> M130/5(CT2)
  [in10] -> M130/6(MR2)
  [in11] -> M130/7(T2)
  [in12] -> M130/8(EB2)
  M130/1(LL1) -> Eval129/1(In1)
  M130/2(LL2) -> Eval129/2(In2)
  Eval129/1(Out1) -> To Workspace129/1
  [in1] -> M131/1(CT1)
  [in4] -> M131/2(MR1)
  [in5] -> M131/3(T1)
  [in6] -> M131/4(EB1)
  [in7] -> M131/5(CT2)
  [in10] -> M131/6(MR2)
  [in11] -> M131/7(T2)
  [in12] -> M131/8(EB2)
  M131/1(LL1) -> Eval130/1(In1)
  M131/2(LL2) -> Eval130/2(In2)
  Eval130/1(Out1) -> To Workspace130/1
  [in1] -> M132/1(CT1)
  [in4] -> M132/2(MR1)
  [in5] -> M132/3(T1)
  [in6] -> M132/4(EB1)
  [in7] -> M132/5(CT2)
  [in10] -> M132/6(MR2)
  [in11] -> M132/7(T2)
  [in12] -> M132/8(EB2)
  M132/1(LL1) -> Eval131/1(In1)
  M132/2(LL2) -> Eval131/2(In2)
  Eval131/1(Out1) -> To Workspace131/1
  [in1] -> M133/1(CT1)
  [in4] -> M133/2(MR1)
  [in5] -> M133/3(T1)
  [in6] -> M133/4(EB1)
  [in7] -> M133/5(CT2)
  [in10] -> M133/6(MR2)
  [in11] -> M133/7(T2)
  [in12] -> M133/8(EB2)
  M133/1(LL1) -> Eval132/1(In1)
  M133/2(LL2) -> Eval132/2(In2)
  Eval132/1(Out1) -> To Workspace132/1
  [in1] -> M134/1(CT1)
  [in4] -> M134/2(MR1)
  [in5] -> M134/3(T1)
  [in6] -> M134/4(EB1)
  [in7] -> M134/5(CT2)
  [in10] -> M134/6(MR2)
  [in11] -> M134/7(T2)
  [in12] -> M134/8(EB2)
  M134/1(LL1) -> Eval133/1(In1)
  M134/2(LL2) -> Eval133/2(In2)
  Eval133/1(Out1) -> To Workspace133/1
  [in1] -> M135/1(CT1)
  [in4] -> M135/2(MR1)
  [in5] -> M135/3(T1)
  [in6] -> M135/4(EB1)
  [in7] -> M135/5(CT2)
  [in10] -> M135/6(MR2)
  [in11] -> M135/7(T2)
  [in12] -> M135/8(EB2)
  M135/1(LL1) -> Eval134/1(In1)
  M135/2(LL2) -> Eval134/2(In2)
  Eval134/1(Out1) -> To Workspace134/1
  [in1] -> M136/1(CT1)
  [in4] -> M136/2(MR1)
  [in5] -> M136/3(T1)
  [in6] -> M136/4(EB1)
  [in7] -> M136/5(CT2)
  [in10] -> M136/6(MR2)
  [in11] -> M136/7(T2)
  [in12] -> M136/8(EB2)
  M136/1(LL1) -> Eval135/1(In1)
  M136/2(LL2) -> Eval135/2(In2)
  Eval135/1(Out1) -> To Workspace135/1
  [in1] -> M137/1(CT1)
  [in4] -> M137/2(MR1)
  [in5] -> M137/3(T1)
  [in6] -> M137/4(EB1)
  [in7] -> M137/5(CT2)
  [in10] -> M137/6(MR2)
  [in11] -> M137/7(T2)
  [in12] -> M137/8(EB2)
  M137/1(LL1) -> Eval136/1(In1)
  M137/2(LL2) -> Eval136/2(In2)
  Eval136/1(Out1) -> To Workspace136/1
  [in1] -> M138/1(CT1)
  [in4] -> M138/2(MR1)
  [in5] -> M138/3(T1)
  [in6] -> M138/4(EB1)
  [in7] -> M138/5(CT2)
  [in10] -> M138/6(MR2)
  [in11] -> M138/7(T2)
  [in12] -> M138/8(EB2)
  M138/1(LL1) -> Eval137/1(In1)
  M138/2(LL2) -> Eval137/2(In2)
  Eval137/1(Out1) -> To Workspace137/1
  [in1] -> M140/1(CT1)
  [in4] -> M140/2(MR1)
  [in5] -> M140/3(T1)
  [in6] -> M140/4(EB1)
  [in7] -> M140/5(CT2)
  [in10] -> M140/6(MR2)
  [in11] -> M140/7(T2)
  [in12] -> M140/8(EB2)
  M140/1(LL1) -> Eval139/1(In1)
  M140/2(LL2) -> Eval139/2(In2)
  Eval139/1(Out1) -> To Workspace139/1
  [in1] -> M141/1(CT1)
  [in4] -> M141/2(MR1)
  [in5] -> M141/3(T1)
  [in6] -> M141/4(EB1)
  [in7] -> M141/5(CT2)
  [in10] -> M141/6(MR2)
  [in11] -> M141/7(T2)
  [in12] -> M141/8(EB2)
  M141/1(LL1) -> Eval140/1(In1)
  M141/2(LL2) -> Eval140/2(In2)
  Eval140/1(Out1) -> To Workspace140/1
  [in1] -> M142/1(CT1)
  [in4] -> M142/2(MR1)
  [in5] -> M142/3(T1)
  [in6] -> M142/4(EB1)
  [in7] -> M142/5(CT2)
  [in10] -> M142/6(MR2)
  [in11] -> M142/7(T2)
  [in12] -> M142/8(EB2)
  M142/1(LL1) -> Eval141/1(In1)
  M142/2(LL2) -> Eval141/2(In2)
  Eval141/1(Out1) -> To Workspace141/1
  [in1] -> M143/1(CT1)
  [in4] -> M143/2(MR1)
  [in5] -> M143/3(T1)
  [in6] -> M143/4(EB1)
  [in7] -> M143/5(CT2)
  [in10] -> M143/6(MR2)
  [in11] -> M143/7(T2)
  [in12] -> M143/8(EB2)
  M143/1(LL1) -> Eval142/1(In1)
  M143/2(LL2) -> Eval142/2(In2)
  Eval142/1(Out1) -> To Workspace142/1
  [in1] -> M144/1(CT1)
  [in4] -> M144/2(MR1)
  [in5] -> M144/3(T1)
  [in6] -> M144/4(EB1)
  [in7] -> M144/5(CT2)
  [in10] -> M144/6(MR2)
  [in11] -> M144/7(T2)
  [in12] -> M144/8(EB2)
  M144/1(LL1) -> Eval143/1(In1)
  M144/2(LL2) -> Eval143/2(In2)
  Eval143/1(Out1) -> To Workspace143/1
  [in1] -> M145/1(CT1)
  [in4] -> M145/2(MR1)
  [in5] -> M145/3(T1)
  [in6] -> M145/4(EB1)
  [in7] -> M145/5(CT2)
  [in10] -> M145/6(MR2)
  [in11] -> M145/7(T2)
  [in12] -> M145/8(EB2)
  M145/1(LL1) -> Eval144/1(In1)
  M145/2(LL2) -> Eval144/2(In2)
  Eval144/1(Out1) -> To Workspace144/1
  [in1] -> M146/1(CT1)
  [in4] -> M146/2(MR1)
  [in5] -> M146/3(T1)
  [in6] -> M146/4(EB1)
  [in7] -> M146/5(CT2)
  [in10] -> M146/6(MR2)
  [in11] -> M146/7(T2)
  [in12] -> M146/8(EB2)
  M146/1(LL1) -> Eval145/1(In1)
  M146/2(LL2) -> Eval145/2(In2)
  Eval145/1(Out1) -> To Workspace145/1
  [in1] -> M147/1(CT1)
  [in4] -> M147/2(MR1)
  [in5] -> M147/3(T1)
  [in6] -> M147/4(EB1)
  [in7] -> M147/5(CT2)
  [in10] -> M147/6(MR2)
  [in11] -> M147/7(T2)
  [in12] -> M147/8(EB2)
  M147/1(LL1) -> Eval146/1(In1)
  M147/2(LL2) -> Eval146/2(In2)
  Eval146/1(Out1) -> To Workspace146/1
  [in1] -> M148/1(CT1)
  [in4] -> M148/2(MR1)
  [in5] -> M148/3(T1)
  [in6] -> M148/4(EB1)
  [in7] -> M148/5(CT2)
  [in10] -> M148/6(MR2)
  [in11] -> M148/7(T2)
  [in12] -> M148/8(EB2)
  M148/1(LL1) -> Eval147/1(In1)
  M148/2(LL2) -> Eval147/2(In2)
  Eval147/1(Out1) -> To Workspace147/1
  [in1] -> M149/1(CT1)
  [in4] -> M149/2(MR1)
  [in5] -> M149/3(T1)
  [in6] -> M149/4(EB1)
  [in7] -> M149/5(CT2)
  [in10] -> M149/6(MR2)
  [in11] -> M149/7(T2)
  [in12] -> M149/8(EB2)
  M149/1(LL1) -> Eval148/1(In1)
  M149/2(LL2) -> Eval148/2(In2)
  Eval148/1(Out1) -> To Workspace148/1
  [in1] -> M150/1(CT1)
  [in4] -> M150/2(MR1)
  [in5] -> M150/3(T1)
  [in6] -> M150/4(EB1)
  [in7] -> M150/5(CT2)
  [in10] -> M150/6(MR2)
  [in11] -> M150/7(T2)
  [in12] -> M150/8(EB2)
  M150/1(LL1) -> Eval149/1(In1)
  M150/2(LL2) -> Eval149/2(In2)
  Eval149/1(Out1) -> To Workspace149/1
  [in1] -> M151/1(CT1)
  [in4] -> M151/2(MR1)
  [in5] -> M151/3(T1)
  [in6] -> M151/4(EB1)
  [in7] -> M151/5(CT2)
  [in10] -> M151/6(MR2)
  [in11] -> M151/7(T2)
  [in12] -> M151/8(EB2)
  M151/1(LL1) -> Eval150/1(In1)
  M151/2(LL2) -> Eval150/2(In2)
  Eval150/1(Out1) -> To Workspace150/1
  [in1] -> M152/1(CT1)
  [in4] -> M152/2(MR1)
  [in5] -> M152/3(T1)
  [in6] -> M152/4(EB1)
  [in7] -> M152/5(CT2)
  [in10] -> M152/6(MR2)
  [in11] -> M152/7(T2)
  [in12] -> M152/8(EB2)
  M152/1(LL1) -> Eval151/1(In1)
  M152/2(LL2) -> Eval151/2(In2)
  Eval151/1(Out1) -> To Workspace151/1
  [in1] -> M153/1(CT1)
  [in4] -> M153/2(MR1)
  [in5] -> M153/3(T1)
  [in6] -> M153/4(EB1)
  [in7] -> M153/5(CT2)
  [in10] -> M153/6(MR2)
  [in11] -> M153/7(T2)
  [in12] -> M153/8(EB2)
  M153/1(LL1) -> Eval152/1(In1)
  M153/2(LL2) -> Eval152/2(In2)
  Eval152/1(Out1) -> To Workspace152/1
  [in1] -> M154/1(CT1)
  [in4] -> M154/2(MR1)
  [in5] -> M154/3(T1)
  [in6] -> M154/4(EB1)
  [in7] -> M154/5(CT2)
  [in10] -> M154/6(MR2)
  [in11] -> M154/7(T2)
  [in12] -> M154/8(EB2)
  M154/1(LL1) -> Eval153/1(In1)
  M154/2(LL2) -> Eval153/2(In2)
  Eval153/1(Out1) -> To Workspace153/1
  [in1] -> M155/1(CT1)
  [in4] -> M155/2(MR1)
  [in5] -> M155/3(T1)
  [in6] -> M155/4(EB1)
  [in7] -> M155/5(CT2)
  [in10] -> M155/6(MR2)
  [in11] -> M155/7(T2)
  [in12] -> M155/8(EB2)
  M155/1(LL1) -> Eval154/1(In1)
  M155/2(LL2) -> Eval154/2(In2)
  Eval154/1(Out1) -> To Workspace154/1
  [in1] -> M156/1(CT1)
  [in4] -> M156/2(MR1)
  [in5] -> M156/3(T1)
  [in6] -> M156/4(EB1)
  [in7] -> M156/5(CT2)
  [in10] -> M156/6(MR2)
  [in11] -> M156/7(T2)
  [in12] -> M156/8(EB2)
  M156/1(LL1) -> Eval155/1(In1)
  M156/2(LL2) -> Eval155/2(In2)
  Eval155/1(Out1) -> To Workspace155/1
  [in1] -> M157/1(CT1)
  [in4] -> M157/2(MR1)
  [in5] -> M157/3(T1)
  [in6] -> M157/4(EB1)
  [in7] -> M157/5(CT2)
  [in10] -> M157/6(MR2)
  [in11] -> M157/7(T2)
  [in12] -> M157/8(EB2)
  M157/1(LL1) -> Eval156/1(In1)
  M157/2(LL2) -> Eval156/2(In2)
  Eval156/1(Out1) -> To Workspace156/1
  [in1] -> M158/1(CT1)
  [in4] -> M158/2(MR1)
  [in5] -> M158/3(T1)
  [in6] -> M158/4(EB1)
  [in7] -> M158/5(CT2)
  [in10] -> M158/6(MR2)
  [in11] -> M158/7(T2)
  [in12] -> M158/8(EB2)
  M158/1(LL1) -> Eval157/1(In1)
  M158/2(LL2) -> Eval157/2(In2)
  Eval157/1(Out1) -> To Workspace157/1
  [in1] -> M159/1(CT1)
  [in4] -> M159/2(MR1)
  [in5] -> M159/3(T1)
  [in6] -> M159/4(EB1)
  [in7] -> M159/5(CT2)
  [in10] -> M159/6(MR2)
  [in11] -> M159/7(T2)
  [in12] -> M159/8(EB2)
  M159/1(LL1) -> Eval158/1(In1)
  M159/2(LL2) -> Eval158/2(In2)
  Eval158/1(Out1) -> To Workspace158/1
  [in1] -> M160/1(CT1)
  [in4] -> M160/2(MR1)
  [in5] -> M160/3(T1)
  [in6] -> M160/4(EB1)
  [in7] -> M160/5(CT2)
  [in10] -> M160/6(MR2)
  [in11] -> M160/7(T2)
  [in12] -> M160/8(EB2)
  M160/1(LL1) -> Eval159/1(In1)
  M160/2(LL2) -> Eval159/2(In2)
  Eval159/1(Out1) -> To Workspace159/1
  [in1] -> M161/1(CT1)
  [in4] -> M161/2(MR1)
  [in5] -> M161/3(T1)
  [in6] -> M161/4(EB1)
  [in7] -> M161/5(CT2)
  [in10] -> M161/6(MR2)
  [in11] -> M161/7(T2)
  [in12] -> M161/8(EB2)
  M161/1(LL1) -> Eval160/1(In1)
  M161/2(LL2) -> Eval160/2(In2)
  Eval160/1(Out1) -> To Workspace160/1
  [in1] -> M162/1(CT1)
  [in4] -> M162/2(MR1)
  [in5] -> M162/3(T1)
  [in6] -> M162/4(EB1)
  [in7] -> M162/5(CT2)
  [in10] -> M162/6(MR2)
  [in11] -> M162/7(T2)
  [in12] -> M162/8(EB2)
  M162/1(LL1) -> Eval161/1(In1)
  M162/2(LL2) -> Eval161/2(In2)
  Eval161/1(Out1) -> To Workspace161/1
  [in1] -> M163/1(CT1)
  [in4] -> M163/2(MR1)
  [in5] -> M163/3(T1)
  [in6] -> M163/4(EB1)
  [in7] -> M163/5(CT2)
  [in10] -> M163/6(MR2)
  [in11] -> M163/7(T2)
  [in12] -> M163/8(EB2)
  M163/1(LL1) -> Eval162/1(In1)
  M163/2(LL2) -> Eval162/2(In2)
  Eval162/1(Out1) -> To Workspace162/1
  [in1] -> M164/1(CT1)
  [in4] -> M164/2(MR1)
  [in5] -> M164/3(T1)
  [in6] -> M164/4(EB1)
  [in7] -> M164/5(CT2)
  [in10] -> M164/6(MR2)
  [in11] -> M164/7(T2)
  [in12] -> M164/8(EB2)
  M164/1(LL1) -> Eval163/1(In1)
  M164/2(LL2) -> Eval163/2(In2)
  Eval163/1(Out1) -> To Workspace163/1
  [in1] -> M226/1(CT1)
  [in4] -> M226/2(MR1)
  [in5] -> M226/3(T1)
  [in6] -> M226/4(EB1)
  [in7] -> M226/5(CT2)
  [in10] -> M226/6(MR2)
  [in11] -> M226/7(T2)
  [in12] -> M226/8(EB2)
  M226/1(LL1) -> Eval225/1(In1)
  M226/2(LL2) -> Eval225/2(In2)
  Eval225/1(Out1) -> To Workspace225/1
  [in1] -> M227/1(CT1)
  [in4] -> M227/2(MR1)
  [in5] -> M227/3(T1)
  [in6] -> M227/4(EB1)
  [in7] -> M227/5(CT2)
  [in10] -> M227/6(MR2)
  [in11] -> M227/7(T2)
  [in12] -> M227/8(EB2)
  M227/1(LL1) -> Eval226/1(In1)
  M227/2(LL2) -> Eval226/2(In2)
  Eval226/1(Out1) -> To Workspace226/1
  [in1] -> M228/1(CT1)
  [in4] -> M228/2(MR1)
  [in5] -> M228/3(T1)
  [in6] -> M228/4(EB1)
  [in7] -> M228/5(CT2)
  [in10] -> M228/6(MR2)
  [in11] -> M228/7(T2)
  [in12] -> M228/8(EB2)
  M228/1(LL1) -> Eval227/1(In1)
  M228/2(LL2) -> Eval227/2(In2)
  Eval227/1(Out1) -> To Workspace227/1
  [in1] -> M229/1(CT1)
  [in4] -> M229/2(MR1)
  [in5] -> M229/3(T1)
  [in6] -> M229/4(EB1)
  [in7] -> M229/5(CT2)
  [in10] -> M229/6(MR2)
  [in11] -> M229/7(T2)
  [in12] -> M229/8(EB2)
  M229/1(LL1) -> Eval228/1(In1)
  M229/2(LL2) -> Eval228/2(In2)
  Eval228/1(Out1) -> To Workspace228/1
  [in1] -> M230/1(CT1)
  [in4] -> M230/2(MR1)
  [in5] -> M230/3(T1)
  [in6] -> M230/4(EB1)
  [in7] -> M230/5(CT2)
  [in10] -> M230/6(MR2)
  [in11] -> M230/7(T2)
  [in12] -> M230/8(EB2)
  M230/1(LL1) -> Eval229/1(In1)
  M230/2(LL2) -> Eval229/2(In2)
  Eval229/1(Out1) -> To Workspace229/1
  Inputs/1(CT1) -> dtc_CT1/1
  dtc_CT1/1 -> CPSUT/1(CT1), [in1]
  Inputs/2(MR1) -> dtc_MR1/1
  dtc_MR1/1 -> CPSUT/2(MR1), [in4]
  Inputs/3(T1) -> dtc_T1/1
  dtc_T1/1 -> CPSUT/3(T1), [in5]
  Inputs/4(EB1) -> dtc_EB1/1
  dtc_EB1/1 -> CPSUT/4(EB1), [in6]
  Inputs/5(CT2) -> dtc_CT2/1
  dtc_CT2/1 -> CPSUT/5(CT2), [in7]
  Inputs/6(MR2) -> dtc_MR2/1
  dtc_MR2/1 -> CPSUT/6(MR2), [in10]
  Inputs/7(T2) -> dtc_T2/1
  dtc_T2/1 -> CPSUT/7(T2), [in11]
  Inputs/8(EB2) -> dtc_EB2/1
  dtc_EB2/1 -> CPSUT/8(EB2), [in12]

== system c00009M_harness/CPSUT ==
  note: VALUES
      | ---------------------------------
      | ControlType = 1 | 2 | 3
      | FillTank = 0 | 1
      | EmptyTank = 0 | 1
      | ManualReference between 0 and 1
      | Tempreature between 0 and 100
      | EmergencyButton = 0 | 1
      | LiquidLevel between 0 and 1 (hmax)
  note: Inputs For Tank2
  note: NAMES
      | --------------------------------------------
      | CT1 = ControlType Tank 1
      | F1 = Fill Tank 1
      | E1 = Empty Tank 1
      | MR1 = Manual Reference Tank1
      | T1 = Temperature Tank 1
      | EB1 = Emergency Button Tank 1
      | LL1 = Liquid Level 1
  note: Inputs For Tank3
  note: Inputs For Tank1
  CT1 : Inport
  MR1 : Inport  Port=2
  T1 : Inport  Port=3
  EB1 : Inport  Port=4
  CT2 : Inport  Port=5
  MR2 : Inport  Port=6
  T2 : Inport  Port=7
  EB2 : Inport  Port=8
  Tank1 : Subsystem
  Tank2 : Subsystem
  LL1 : Outport
  LL2 : Outport  Port=2
  wires:
  EB1/1 -> Tank1/4(EB1)
  Tank2/1(LL2) -> LL2/1, Tank1/5(LL2)
  EB2/1 -> Tank2/4(EB2)
  CT2/1 -> Tank2/1(CT2)
  MR1/1 -> Tank1/2(MR1)
  T1/1 -> Tank1/3(T1)
  Tank1/1(LL1) -> LL1/1, Tank2/5(LL1)
  T2/1 -> Tank2/3(T2)
  CT1/1 -> Tank1/1(CT1)
  MR2/1 -> Tank2/2(MR2)

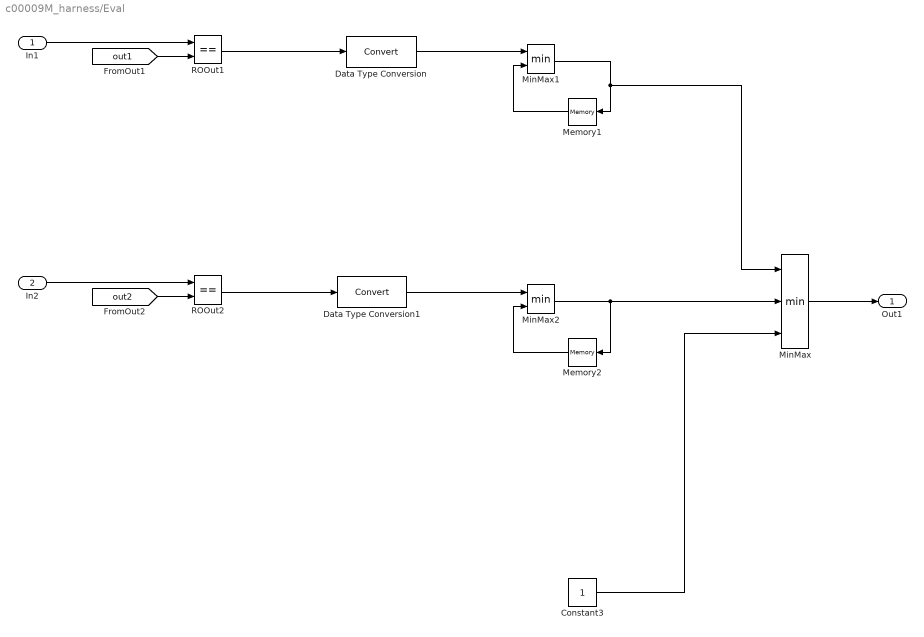
== system c00009M_harness/Eval ==
  In1 : Inport
  In2 : Inport  Port=2
  Constant3 : Constant
  Data Type Conversion : DataTypeConversion
  Data Type Conversion1 : DataTypeConversion
  Memory1 : Memory  InitialCondition=1
  Memory2 : Memory  InitialCondition=1
  MinMax : MinMax  Inputs=3
  MinMax1 : MinMax  Inputs=2
  MinMax2 : MinMax  Inputs=2
  ROOut1 : RelationalOperator  Operator===  OutDataTypeStr=boolean  RndMeth=Simplest
  ROOut2 : RelationalOperator  Operator===  OutDataTypeStr=boolean  RndMeth=Simplest
  Out1 : Outport
  wires:
  MinMax/1 -> Out1/1
  [out1] -> ROOut1/2
  In2/1 -> ROOut2/1
  In1/1 -> ROOut1/1
  [out2] -> ROOut2/2
  Memory1/1 -> MinMax1/2
  ROOut2/1 -> Data Type Conversion1/1
  Memory2/1 -> MinMax2/2
  ROOut1/1 -> Data Type Conversion/1
  MinMax2/1 -> Memory2/1, MinMax/2
  MinMax1/1 -> MinMax/1, Memory1/1
  Data Type Conversion/1 -> MinMax1/1
  Data Type Conversion1/1 -> MinMax2/1
  Constant3/1 -> MinMax/3

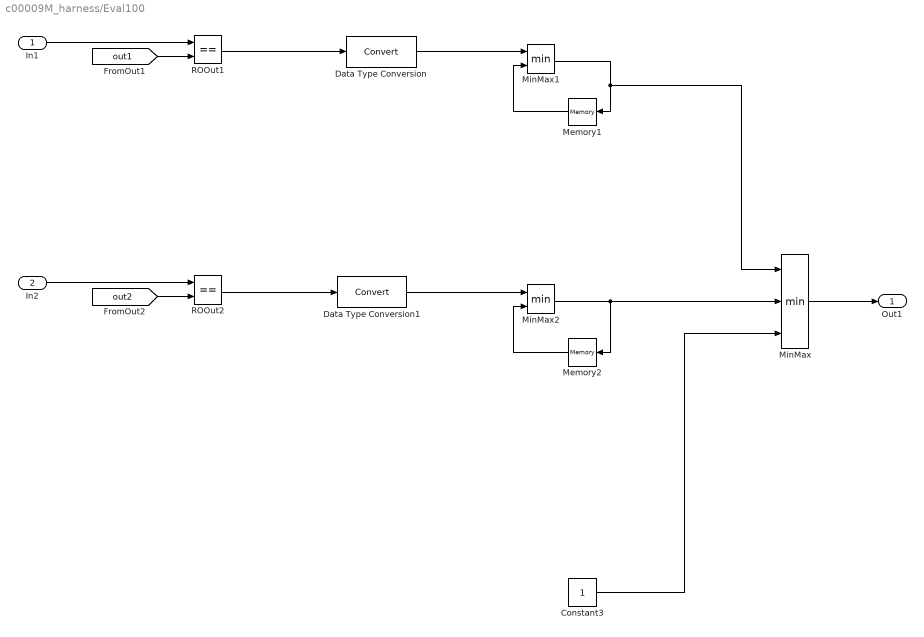
== system c00009M_harness/Eval100 ==
  In1 : Inport
  In2 : Inport  Port=2
  Constant3 : Constant
  Data Type Conversion : DataTypeConversion
  Data Type Conversion1 : DataTypeConversion
  Memory1 : Memory  InitialCondition=1
  Memory2 : Memory  InitialCondition=1
  MinMax : MinMax  Inputs=3
  MinMax1 : MinMax  Inputs=2
  MinMax2 : MinMax  Inputs=2
  ROOut1 : RelationalOperator  Operator===  OutDataTypeStr=boolean  RndMeth=Simplest
  ROOut2 : RelationalOperator  Operator===  OutDataTypeStr=boolean  RndMeth=Simplest
  Out1 : Outport
  wires:
  Data Type Conversion1/1 -> MinMax2/1
  Data Type Conversion/1 -> MinMax1/1
  MinMax1/1 -> Memory1/1, MinMax/1
  MinMax2/1 -> MinMax/2, Memory2/1
  ROOut1/1 -> Data Type Conversion/1
  Memory2/1 -> MinMax2/2
  ROOut2/1 -> Data Type Conversion1/1
  Memory1/1 -> MinMax1/2
  [out2] -> ROOut2/2
  In1/1 -> ROOut1/1
  In2/1 -> ROOut2/1
  [out1] -> ROOut1/2
  MinMax/1 -> Out1/1
  Constant3/1 -> MinMax/3

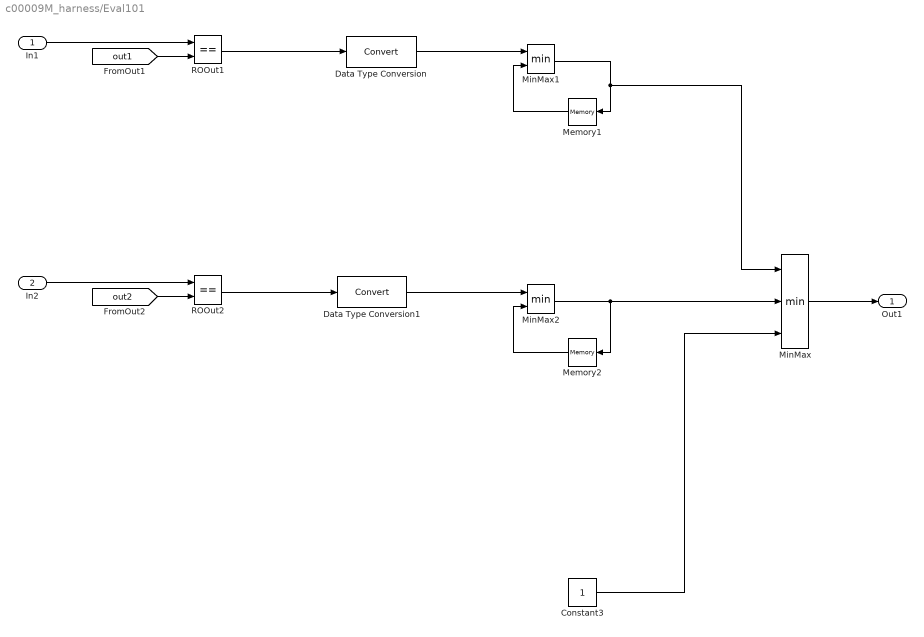
== system c00009M_harness/Eval101 ==
  In1 : Inport
  In2 : Inport  Port=2
  Constant3 : Constant
  Data Type Conversion : DataTypeConversion
  Data Type Conversion1 : DataTypeConversion
  Memory1 : Memory  InitialCondition=1
  Memory2 : Memory  InitialCondition=1
  MinMax : MinMax  Inputs=3
  MinMax1 : MinMax  Inputs=2
  MinMax2 : MinMax  Inputs=2
  ROOut1 : RelationalOperator  Operator===  OutDataTypeStr=boolean  RndMeth=Simplest
  ROOut2 : RelationalOperator  Operator===  OutDataTypeStr=boolean  RndMeth=Simplest
  Out1 : Outport
  wires:
  Data Type Conversion1/1 -> MinMax2/1
  Data Type Conversion/1 -> MinMax1/1
  MinMax1/1 -> Memory1/1, MinMax/1
  MinMax2/1 -> MinMax/2, Memory2/1
  ROOut1/1 -> Data Type Conversion/1
  Memory2/1 -> MinMax2/2
  ROOut2/1 -> Data Type Conversion1/1
  Memory1/1 -> MinMax1/2
  [out2] -> ROOut2/2
  In1/1 -> ROOut1/1
  In2/1 -> ROOut2/1
  [out1] -> ROOut1/2
  MinMax/1 -> Out1/1
  Constant3/1 -> MinMax/3
